simulink model "Bai24"  (R2015a)
settings: Solver=ode45  StartTime=0.0  StopTime=10.0  RelTol=1e-3
settings Model: Creator=Win 10  LastModifiedBy=Win 10

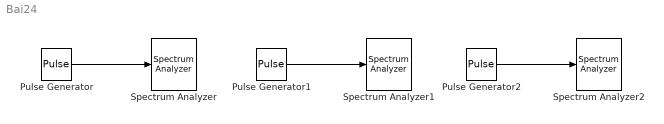
== system Bai24 ==
  Pulse Generator : DiscretePulseGenerator  Amplitude=3  Period=100  PulseWidth=2  PhaseDelay=1  SampleTime=1/10000  VectorParams1D=off
  Pulse Generator1 : DiscretePulseGenerator  PulseType=Time based  Amplitude=3  Period=0.5  PulseWidth=25  PhaseDelay=1  SampleTime=1/1000  VectorParams1D=off
  Pulse Generator2 : DiscretePulseGenerator  PulseType=Time based  Amplitude=3  Period=0.5  PulseWidth=50  PhaseDelay=1  SampleTime=1/1000  VectorParams1D=off
  Spectrum Analyzer : SpectrumAnalyzer
  Spectrum Analyzer1 : SpectrumAnalyzer
  Spectrum Analyzer2 : SpectrumAnalyzer
  wires:
  Pulse Generator/1 -> Spectrum Analyzer/1
  Pulse Generator1/1 -> Spectrum Analyzer1/1
  Pulse Generator2/1 -> Spectrum Analyzer2/1
